simulink model "TargetPosVel"  (R2024b)
settings: Solver=ode4  StartTime=0.0  StopTime=stopTime  FixedStep=timeStep  RelTol=1e-3
values from neighbouring files (symbols this model uses):
  c = 299792458    [FMC.m]
  CD = 2.2    [FMC.m]
  dayValue = 1    [FMC.m]    (also in validation.m)
  dimx = 226.3/1000    (= 0.2263)    [FMC.m]
  dimz = 360/1000    (= 0.36)    [FMC.m]
  FL = 50e-3    (= 0.05)    [FMC.m]
  fps = 1/timeStep    (= 20)    [FMC.m]
  hourValue = 12    [FMC.m]    (also in validation.m)
  I = [Ixx Ixy Ixz; Ixy Iyy Iyz; Ixz Iyz Izz]    [FMC.m]
  I_W = [I_w 0 0; 0 I_w 0; 0 0 I_w]    [FMC.m]
  kd = 0.022    [FMC.m]
  kq = 0.0032    [FMC.m]
  L_pixel = 4.8e-6    (= 4.8e-06)    [FMC.m]
  max_h = I_w*max_speed    (= 0.00954258768528)    [FMC.m]
  max_t = 2e-3    (= 0.002)    [FMC.m]
  minuteValue = 0    [FMC.m]    (also in validation.m)
  mu_E = 3.986004418e14    (= 398600441800000)    [FMC.m]
  Omega_E = 7.2921159e-5    (= 7.2921159e-05)    [FMC.m]
  P0_Kfilter = blkdiag(eye(3), eye(3))    [FMC.m]
  Phi = 1358    [FMC.m]
  pointing_body = [0,0,1]    [FMC.m]
  q = 0.6    [FMC.m]
  Q_b = 0.05*eye(3)    [FMC.m]
  Q_LoS = 0.1*eye(3)    [FMC.m]
  quat0 = [0.6387; -0.3737; 0.6003; 0.3034]    [FMC.m]
  R_E = 6378*1000    (= 6378000)    [FMC.m]
  R_meas = norm(LoS_0)*L_pixel*fps/FL*Q_b    [FMC.m]
  rand_vec = rand_vec/norm(rand_vec)    [FMC.m]
  rcp = [0.013 0.02 0.05]    [FMC.m]
  res_dipole = 0.05    [FMC.m]
  secondValue = 0    [FMC.m]    (also in validation.m)
  sma = R_E + H    (= 6628000)    [FMC.m]
  timeStep = 0.05    [FMC.m]
  w0 = [w0x; w0y; w0z]    [FMC.m]
  x0_Kfilter = [LoS_0,;b_0]    [FMC.m]
  yearValue = 2025    [FMC.m]    (also in validation.m)
undefined symbols (not defined in the file or in its folder): IAU, WMM2020
libraries: aerolibtransform2 x14, aerolibutil x13, matrix_library x12, vrlib x5, sharedtransform x2, sharedTrackingLibrary x1, aerolibatmos2 x1, aerolibgravity2 x1, sensorgpslib x1, visionsources x1
(part 2 of 2)

== matlab function TargetPosVel/Target Velocity and Position/Subsystem1/Subsystem4/MATLAB Function1 ==
  data: frame1 input size=[1200,1920,3]; u_est output size=1; frame2 input size=[1200,1920,3]; v_est output size=1; precFactor input
function [u_est, v_est] = motion_estimation(frame1, frame2, precFactor)

% Motion estimation between two frames through cross correlation. This code
% gives the same precision as the FFT upsampled cross correlation in a
% small fraction of the computation time and with reduced memory 
% requirements. It obtains an initial estimate of the crosscorrelation peak
% by an FFT and then refines the shift estimation by upsampling the DFT
% only in a small neighborhood of that estimate by means of a 
% matrix-multiply DFT. With this procedure all the image points are used to
% compute the upsampled crosscorrelation.

%% Preprocessing
f = im2single(im2gray(frame1));
g = im2single(im2gray(frame2));

% winRows    = 240;
% winCols    = 384;
% windowSize = [winRows, winCols];
% C          = SelectRegionEdges(f, windowSize);
% 
% f = im2single(f(C(1):C(1)+winRows-1, C(2):C(2)+winCols-1));
% g = im2single(g(C(1):C(1)+winRows-1, C(2):C(2)+winCols-1));

H1 = hann(size((f), 1));
H2 = hann(size((f), 2));

hannWindow = H1*H2';

f = f.*hannWindow;
g = g.*hannWindow;

img1ft = fft2(f);
img2ft = fft2(g);

%% Start with precFactor == 1 to get an integer shift between images
[nr, nc] = size(f);

Nr = ifftshift(-fix(nr/2):ceil(nr/2)-1);
Nc = ifftshift(-fix(nc/2):ceil(nc/2)-1);

% Calculate the cross correlation function between the two images
crossCorr    = ifft2((img2ft.*conj(img1ft))./abs(img2ft.*conj(img1ft)));
abscrossCorr = abs(crossCorr);

[~, maxIndex] = max(abscrossCorr(:)); % linear index of max
[row_shift, col_shift] = ind2sub(size(abscrossCorr), maxIndex);

% Change shifts so that they represent relative shifts and not indices
row_shift = Nr(row_shift);
col_shift = Nc(col_shift);

%% If precision factor is higher than 1, proceed with subpixel refinement
if precFactor >= 2
    %%% DFT computation %%%
    % Center of output array at dftshift+1
    dftshift = fix(ceil(precFactor*1.5)/2);

    % Matrix multiply DFT around the current shift estimate
    crossCorr = conj(dftups((img1ft.*conj(img2ft)), ...
                            ceil(precFactor*1.5), ...
                            ceil(precFactor*1.5), ...
                            precFactor, ...
                            dftshift - row_shift*precFactor, ...
                            dftshift - col_shift*precFactor));

    % Locate maximum and map back to original pixel grid 
    abscrossCorr = abs(crossCorr);

    [~, maxIndex] = max(abscrossCorr(:));       % linear index of max
    [rloc, cloc] = ind2sub(size(abscrossCorr), maxIndex);
    rloc         = rloc - dftshift - 1;
    cloc         = cloc - dftshift - 1;
    
    % Divide rloc and cloc by precFactor to get back to original unit pixel
    % dimensions and sum to the initial integer estimate
    row_shift = row_shift + rloc/precFactor;
    col_shift = col_shift + cloc/precFactor;
end

%% Image final shifts
u_est = col_shift;
v_est = row_shift;

end

%% Fourier Transform Up-sampling
function out = dftups(in, nor, noc, precFactor, roff, coff)

% Upsampled DFT by matrix multiplies, can compute an upsampled DFT in just
% a small region.
% 
% Inputs:
% - precFactor: Precision factor.
% - nor, noc:   Number of pixels in the output upsampled DFT, in units of 
%               upsampled pixels.
% - roff, coff: Row and column offsets, allow to shift the output array to
%               a region of interest on the DFT.
%
% Receives DC in upper left corner, image center must be in (1, 1) 
%
% This code is intended to provide the same result as if the following
% operations were performed:
%
%   1. Embed the array in an array that is 'precFactor' times larger in 
%      each dimension. ifftshift to bring the center of the image to (1,1).
%   2. Take the FFT of the larger array
%   3. Extract an [nor, noc] region of the result. Starting with the 
%      [roff+1 coff+1] element.
%
% It achieves this result by computing the DFT in the output array without
% the need to zeropad. Much faster and memory efficient than the 
% zero-padded  FFT approach if [nor, noc] are much smaller than 
% [nr*usfac, nc*usfac]

[nr, nc] = size(in);

% Compute kernels and obtain DFT by matrix products
kernc = exp((-1i*2*pi/(nc*precFactor))*(ifftshift(0:nc-1).' - floor(nc/2) )*((0:noc-1) - coff));
kernr = exp((-1i*2*pi/(nr*precFactor))*((0:nor-1).' - roff)*(ifftshift(0:nr-1) - floor(nr/2)));

out = kernr*in*kernc;

end

% %% Select region of interest based on number of edges in the image
% function TopLeftAngle = SelectRegionEdges(img, windowSize)
% 
% edgeMap = edge(img, 'Canny');
% 
% windowRows = windowSize(1);
% windowCols = windowSize(2);
% 
% [imgRows, imgCols] = size(img);
% 
% % Region top left angle in the original image (initialization)
% TopLeftAngle = [1, 1];
% 
% % Edge density initialization
% maxDensity = 0;
% 
% for i = 1:windowRows/2:imgRows - windowRows
%     for j = 1:windowCols/2:imgCols - windowCols
%         % Extract the current window
%         Window = edgeMap(i:i+windowRows-1, j:j+windowCols-1);
% 
%         % Find number of edges in the selected region
%         edgeDensity = sum(Window(:));
% 
%         % Update the region center if the new value is higher than the 
%         % previous computed one
%         if edgeDensity > maxDensity
%             maxDensity = edgeDensity;
%             TopLeftAngle = [i, j];
% 
%         end
%     end
% end
% end

== matlab function TargetPosVel/Main/Subsystem/Quaternion kinematics/MATLAB Function ==
  data: omega input; OMEGA output
function OMEGA = buildMatrix(omega)

OMEGA = [   0      -omega(1)  -omega(2)  -omega(3);
         omega(1)      0       omega(3)  -omega(2);
         omega(2)  -omega(3)      0       omega(1);
         omega(3)   omega(2)  -omega(1)      0    ];

end

== matlab function TargetPosVel/MATLAB Function ==
  data: u input; x0_new output; v input; dt input; x0 input; P0 input; P0_new output; f input; Lpix input; r_sat input; v_sat input; omega_b input; Q_b input; Q_LoS input; q_eci2cam input size=[4,1]; R_meas input
function [x0_new, P0_new] = ekf_lineofsight(u, v, dt, x0, P0, f, Lpix, ...
                                            r_sat, v_sat, omega_b, Q_b, ...
                                            Q_LoS, q_eci2cam, R_meas)


%% Set-up
fps          = 1/dt;
los_eci_prev = x0(1:3);
los_eci_prev = reshape(los_eci_prev, [], 1);
b_OF_prev    = x0(4:6);
b_OF_prev    = reshape(b_OF_prev, [], 1);
Qsys         = blkdiag(Q_LoS, Q_b);
R_cam        = quat2dcm(reshape(q_eci2cam, 1, []));
omega_cam    = reshape(omega_b, [], 1);
z_meas       = [u; v; 0];
r_sat        = reshape(r_sat, [], 1);
v_sat        = reshape(v_sat, [], 1);

%% Compute measurement Jacobian (B in the note)
rho        = norm(los_eci_prev);
omega_skew = skew(R_cam'*omega_cam);
num        = rho^2*(v_sat + omega_skew'*r_sat);
num2       = (v_sat + omega_skew'*r_sat)*(2*los_eci_prev*(r_sat'*los_eci_prev) - rho^2*r_sat)'; 
denom      = r_sat'*los_eci_prev + rho^2; 
r_tar_dot  = v_sat + omega_skew*los_eci_prev - num/denom;

A = omega_skew - num2/denom;
B = f/(fps*Lpix*rho^2)*R_cam*(rho*A - 2*los_eci_prev*r_tar_dot');

%% Construct H
H = [B, eye(3)];

%% Kalman gain
K = P0*H'*inv(H*P0*H' + R_meas);

%% Filter update
h_x_prev = f/(fps*Lpix*rho)*R_cam*(r_tar_dot) + b_OF_prev;
x_new    = [los_eci_prev; b_OF_prev] + K*(z_meas - h_x_prev);

los_eci_new = x_new(1:3);
b_OF_new    = x_new(4:6);

P_new = (eye(6) - K*H)*P0;

%% Compute state transition matrix
rho    = norm(los_eci_new);
num3   = (v_sat + omega_skew'*r_sat)*(2*los_eci_new*(r_sat'*los_eci_new) - rho^2*r_sat)';
denom2 = r_sat'*los_eci_new + rho^2;
A_new  = omega_skew - num3/denom2;
Phi    = blkdiag(eye(3) + A_new*dt, eye(3));

%% Filter propagation
num4        = rho^2*(v_sat + omega_skew'*r_sat);
phi_los_new = omega_skew*los_eci_new - num4/denom2;

x0_new = [phi_los_new; b_OF_new];
P0_new = Phi*P_new*Phi' + Qsys;

end

function S = skew(v)
% Creates skew-symmetric matrix from vector v

S = [  0   -v(3)  v(2);
      v(3)   0   -v(1);
     -v(2)  v(1)   0  ];

end

== matlab function TargetPosVel/Main/Subsystem/GPS/Subsystem1/MATLAB Function ==
  data: jd input; DCM_eci2ecef output
function DCM_eci2ecef = eci2ecef(jd)

% Compute GMST (Greenwich Mean Sidereal Time)
% T = (jd - 2451545.0) / 36525; % Julian centuries from J2000.0
GMST  = mod(280.46061837 + 360.98564736629*(jd - 2451545.0), 360);
theta = deg2rad(GMST); % convert to radians

% Build DCM
DCM_eci2ecef = [ cos(theta),  sin(theta),  0;
                -sin(theta),  cos(theta),  0;
                          0,           0,  1];

end
